simulink model "kut_systeem"  (R2021a)
settings: Solver=FixedStepAuto  StartTime=0.0  StopTime=10  FixedStep=0.001  MaxStep=0.05  MinStep=0.05  RelTol=1e-3
settings Model: Creator=marnixmeersman  LastModifiedBy=trist
settings SolverCC: InitialStep=0.05

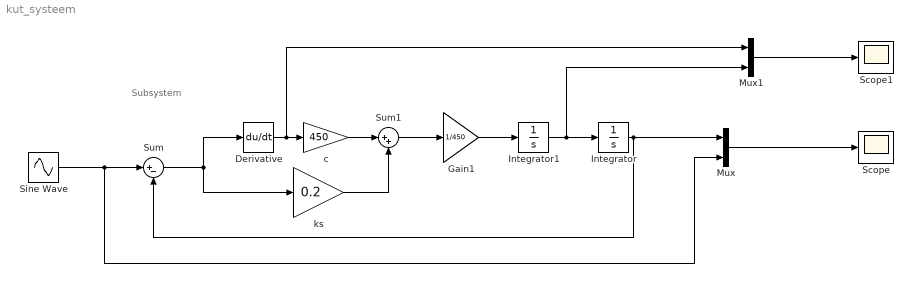
== system kut_systeem ==
  note: Subsystem
  Derivative : Derivative
  Gain1 : Gain  Gain=1/450
  Integrator : Integrator
  Integrator1 : Integrator
  Mux : Mux  Inputs=2
  Mux1 : Mux  Inputs=2
  Scope : Scope
  Scope1 : Scope
  Sine Wave : Sin  Amplitude=0.02  Frequency=8  SampleTime=0
  Sum : Sum  Inputs=|+-
  Sum1 : Sum  Inputs=|++
  c : Gain  Gain=450
  ks : Gain  Gain=0.2
  wires:
  Mux/1 -> Scope/1
  Integrator/1 -> Sum/2, Mux/1
  Sine Wave/1 -> Sum/1, Mux/2
  c/1 -> Sum1/1
  Derivative/1 -> Mux1/1, c/1
  Integrator1/1 -> Mux1/2, Integrator/1
  Sum1/1 -> Gain1/1
  ks/1 -> Sum1/2
  Sum/1 -> ks/1, Derivative/1
  Gain1/1 -> Integrator1/1
  Mux1/1 -> Scope1/1
